simulink model "CoETS_TSEACo"  (R2016b)
settings: configuration reference "CodeGenConfigSet" (kept outside this file)
values from neighbouring files (symbols this model uses):
  CoETS_ctEngEmgcyRunCnt_C = Calibration.Parameter    [init_CoETS_TSEACo.m]
  CoETS_nTSCRmpSlopeNeg_C = Calibration.Parameter    [init_CoETS_TSEACo.m]
  CoETS_nTSCRmpSlopePos_C = Calibration.Parameter    [init_CoETS_TSEACo.m]
  CoETS_numTSEAPrioAE_C = Calibration.Parameter    [init_CoETS_TSEACo.m]
  CoETS_numTSEAPrioDE_C = Calibration.Parameter    [init_CoETS_TSEACo.m]
  CoETS_numTSEAPrioGpsLim_C = Calibration.Parameter    [init_CoETS_TSEACo.m]
  CoETS_numTSEAPrioPE_C = Calibration.Parameter    [init_CoETS_TSEACo.m]
  CoETS_numTSEAPrioTE_C = Calibration.Parameter    [init_CoETS_TSEACo.m]
  CoETS_numTSEAPrioVE_C = Calibration.Parameter    [init_CoETS_TSEACo.m]
  CoETS_stEngEmgcyRunEN_C = Calibration.Parameter    [init_CoETS_TSEACo.m]
  CoETS_stStartRelayCtrl_C = Calibration.Parameter    [init_CoETS_TSEACo.m]
  CoETS_stTboxUse_C = Calibration.Parameter    [init_CoETS_TSEACo.m]
  CoETS_stTSEATrqSpd_C = Calibration.Parameter    [init_CoETS_TSEACo.m]
  CoETS_swtTempSel_C = Calibration.Parameter    [init_CoETS_TSEACo.m]
  CoETS_tEngEmgcyRunTemp_C = Calibration.Parameter    [init_CoETS_TSEACo.m]
  CoETS_tiEngEmgcyRunTime_C = Calibration.Parameter    [init_CoETS_TSEACo.m]
  CoETS_tiEngEmgcyStartTime_C = Calibration.Parameter    [init_CoETS_TSEACo.m]
  CoETS_tiEngLockTime_C = Calibration.Parameter    [init_CoETS_TSEACo.m]
  CoETS_tiSetTimeTSEReq_CUR = Calibration.Parameter    [init_CoETS_TSEACo.m]
  CoETS_tiSetTimeTSEReq_CURX = Calibration.Parameter    [init_CoETS_TSEACo.m]
  CoETS_TrqTSCRmpSlopeNeg_C = Calibration.Parameter    [init_CoETS_TSEACo.m]
  CoETS_TrqTSCRmpSlopePos_C = Calibration.Parameter    [init_CoETS_TSEACo.m]
  Ecu_stGps_Status_C = Calibration.Parameter    [init_CoETS_TSEACo.m]
  EngPrt_nRateSp_C = Calibration.Parameter    [init_CoETS_TSEACo.m]
  Gps_nSpdLmt_C = Calibration.Parameter    [init_CoETS_TSEACo.m]
  TSC_nAEDes_C = Calibration.Parameter    [init_CoETS_TSEACo.m]
  TSC_nDEDes_C = Calibration.Parameter    [init_CoETS_TSEACo.m]
  TSC_nPEDes_C = Calibration.Parameter    [init_CoETS_TSEACo.m]
  TSC_nTEDes_C = Calibration.Parameter    [init_CoETS_TSEACo.m]
  TSC_nVEDes_C = Calibration.Parameter    [init_CoETS_TSEACo.m]
  TSC_rTrqAEDes_C = Calibration.Parameter    [init_CoETS_TSEACo.m]
  TSC_rTrqDEDes_C = Calibration.Parameter    [init_CoETS_TSEACo.m]
  TSC_rTrqPEDes_C = Calibration.Parameter    [init_CoETS_TSEACo.m]
  TSC_rTrqTEDes_C = Calibration.Parameter    [init_CoETS_TSEACo.m]
  TSC_rTrqVEDes_C = Calibration.Parameter    [init_CoETS_TSEACo.m]
  TSC_stAEErr_C = Calibration.Parameter    [init_CoETS_TSEACo.m]
  TSC_stAEMode_C = Calibration.Parameter    [init_CoETS_TSEACo.m]
  TSC_stDEErr_C = Calibration.Parameter    [init_CoETS_TSEACo.m]
  TSC_stDEMode_C = Calibration.Parameter    [init_CoETS_TSEACo.m]
  TSC_stModeBypassEN_C = Calibration.Parameter    [init_CoETS_TSEACo.m]
  TSC_stPEErr_C = Calibration.Parameter    [init_CoETS_TSEACo.m]
  TSC_stPEMode_C = Calibration.Parameter    [init_CoETS_TSEACo.m]
  TSC_stTEErr_C = Calibration.Parameter    [init_CoETS_TSEACo.m]
  TSC_stTEMode_C = Calibration.Parameter    [init_CoETS_TSEACo.m]
  TSC_stVEErr_C = Calibration.Parameter    [init_CoETS_TSEACo.m]
  TSC_stVEMode_C = Calibration.Parameter    [init_CoETS_TSEACo.m]
undefined symbols (not defined in the file or in its folder): CoETS_TSEACo_DT, EngState_conv, HLSDem_KpCorFac_MAPX, Switch_conv, TSC1_stSource_conv
libraries: simulink x82, CXLib x8
(part 1 of 2)
settings Model: Creator=Wollf  LastModifiedBy=xuxingpei
settings ConfigSetRef: SourceLocation=Base Workspace

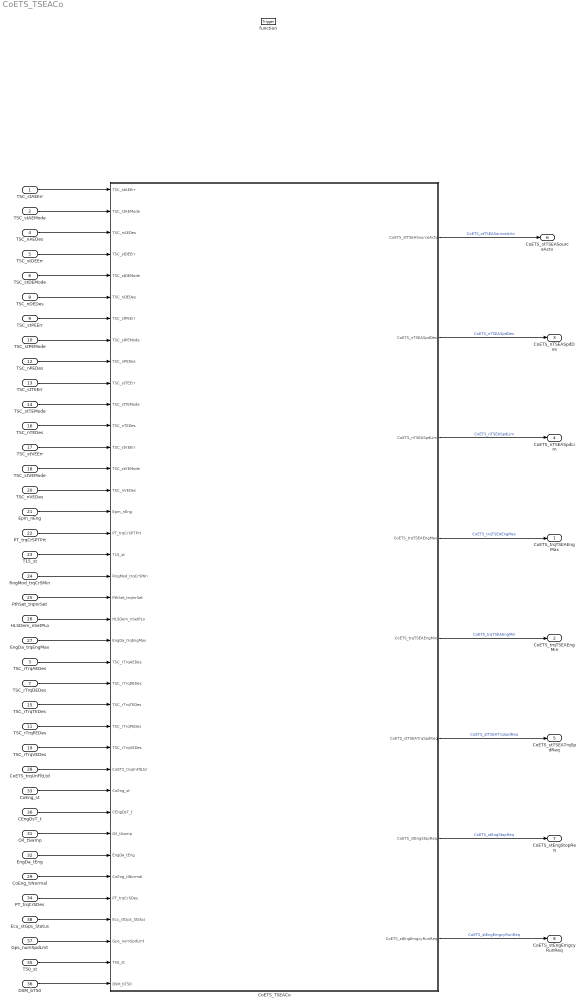
== system CoETS_TSEACo ==
  TSC_stAEErr : Inport  Description=Error status of receiving the TSC1-AE CAN message  OutMin=0  OutMax=1  OutDataTypeStr=State_uint8
  TSC_stAEMode : Inport  Description=Override control mode of TSC1-AE CAN message  Port=2  OutMin=0  OutMax=3  OutDataTypeStr=State_uint8
  TSC_rTrqAEDes : Inport  Description=|  Port=3  OutMin=0  OutMax=125  OutDataTypeStr=State_uint8
      | Requested torque percent / torque limit by TSC1-AE CAN
      | message Nm
  TSC_nAEDes : Inport  Tag=rpm  Description=Requested speed / speed limit by TSC1-AE message  Port=4  OutMin=0  OutMax=6000  OutDataTypeStr=EngSpeed_rpm
  TSC_stDEErr : Inport  Description=Error status of receiving the TSC1-DE CAN message  Port=5  OutMin=0  OutMax=1  OutDataTypeStr=State_uint8
  TSC_stDEMode : Inport  Description=Override control mode of TSC1-DE CAN message  Port=6  OutMin=0  OutMax=3  OutDataTypeStr=State_uint8
  TSC_rTrqDEDes : Inport  Description=|  Port=7  OutMin=0  OutMax=125  OutDataTypeStr=State_uint8
      | Requested torque percent/ torque limit by TSC1-DE CAN
      | message Nm
  TSC_nDEDes : Inport  Tag=rpm  Description=|  Port=8  OutMin=0  OutMax=8000  OutDataTypeStr=EngSpeed_rpm
      | Requested speed / speed limit by TSC1-DE CAN
      | message rpm
  TSC_stPEErr : Inport  Description=Error status of receiving the TSC1-PE CAN message  Port=9  OutMin=0  OutMax=1  OutDataTypeStr=State_uint8
  TSC_stPEMode : Inport  Description=Override control mode of TSC1-PE CAN message  Port=10  OutMin=0  OutMax=3  OutDataTypeStr=State_uint8
  TSC_rTrqPEDes : Inport  Description=|  Port=11  OutMin=0  OutMax=125  OutDataTypeStr=State_uint8
      | Requested torque percent/ torque limit by TSC1-PE CAN
      | message Nm
  TSC_nPEDes : Inport  Tag=rpm  Description=|  Port=12  OutMin=0  OutMax=8000  OutDataTypeStr=EngSpeed_rpm
      | Requested speed / speed limit by TSC1-PE CAN
      | message rpm
  TSC_stTEErr : Inport  Description=Error status of receiving the TSC1-TE CAN message  Port=13  OutMin=0  OutMax=1  OutDataTypeStr=State_uint8
  TSC_stTEMode : Inport  Description=Override control mode of TSC1-TE CAN message  Port=14  OutMin=0  OutMax=3  OutDataTypeStr=State_uint8
  TSC_rTrqTEDes : Inport  Description=|  Port=15  OutMin=0  OutMax=125  OutDataTypeStr=State_uint8
      | Requested torque percent / torque limit by TSC1-TE CAN
      | message Nm
  TSC_nTEDes : Inport  Tag=rpm  Description=|  Port=16  OutMin=0  OutMax=8000  OutDataTypeStr=EngSpeed_rpm
      | Requested speed / speed limit by TSC1-TE CAN
      | message rpm
  TSC_stVEErr : Inport  Description=Error status of receiving the TSC1-VE CAN message  Port=17  OutMin=0  OutMax=1  OutDataTypeStr=State_uint8
  TSC_stVEMode : Inport  Description=Override control mode of TSC1-VE CAN message.  Port=18  OutMin=0  OutMax=3  OutDataTypeStr=State_uint8
  TSC_rTrqVEDes : Inport  Description=|  Port=19  OutMin=0  OutMax=125  OutDataTypeStr=State_uint8
      | Requested torque percent/ torque limit by TSC1-VE CAN
      | message Nm
  TSC_nVEDes : Inport  Tag=rpm  Description=|  Port=20  OutMin=0  OutMax=8000  OutDataTypeStr=EngSpeed_rpm
      | Requested speed / speed limit by TSC1-VE CAN
      | message rpm
  Epm_nEng : Inport  Tag=rpm  Description=Engine speed  Port=21  OutMin=0  OutMax=6000  OutDataTypeStr=EngSpeed_rpm
  PT_trqCrSPTPrt : Inport  Tag=Nm  Description=Application parameter for powertrain protection train protection torque(crankshaft torque)  Port=22  OutMin=-3000  OutMax=3000  OutDataTypeStr=Trq_Nm
  T15_st : Inport  Description=Terminal 15 status after debouncing  Port=23  OutDataTypeStr=Enum: Switch_conv
  RngMod_trqCrSMin : Inport  Tag=Nm  Description=minimal crankshaft torque  Port=24  OutMin=-3276.8  OutMax=3276.7  OutDataTypeStr=Trq_Nm
  PthSet_trqInrSet : Inport  Tag=Nm  Description=Inner torque set value after monitoring limitation  Port=25  OutMin=-3000  OutMax=3276.7  OutDataTypeStr=Trq_Nm
  HLSDem_nSetPLo : Inport  Tag=rpm  Description=Minimum engine speed of HLSDem  Port=26  OutMin=0  OutMax=6000  OutDataTypeStr=EngSpeed_rpm
  EngDa_trqEngMax : Inport  Tag=Nm  Description=Maximum engine output torque  Port=27  OutMin=-3276.8  OutMax=3276.7  OutDataTypeStr=Trq_Nm
  CoETS_trqUnFltLtd : Inport  Tag=Nm  Description=Limited idle speed governor torque  Port=28  OutMin=-3276  OutMax=3276  OutDataTypeStr=Trq_Nm
  CoEng_tiNormal : Inport  Tag=ms  Description="Time since state\"CONENG_RUNNING\"was reached"  Port=29  OutMin=0  OutMax=42949672950  OutDataTypeStr=EngTime_ms
  CEngDsT_t : Inport  Tag=deg  Description=engine coolant temperature after filter  Port=30  OutMin=-200  OutMax=200  OutDataTypeStr=Temp_deg
  Oil_tSwmp : Inport  Tag=deg  Description=Oil temperature in oil sump  Port=31  OutMin=-50  OutMax=200  OutDataTypeStr=Temp_deg
  EngDa_tEng : Inport  Tag=deg  Description=Engine temperature  Port=32  OutMin=-1000  OutMax=1000  OutDataTypeStr=Temp_deg
  CoEng_st : Inport  Description=Engine coordinator state  Port=33  OutDataTypeStr=Enum: EngState_conv
  PT_trqCrSDes : Inport  Tag=Nm  Description=Application parameter for requested propulsion torque to engine(crankshaft torque)  Port=34  OutMin=-3000  OutMax=3000  OutDataTypeStr=Trq_Nm
  T50_st : Inport  Description=Terminal 50 status after debouncing  Port=35  OutDataTypeStr=Enum: Switch_conv
  DSM_bT50 : Inport  Description=DSM status from T50 switch  Port=36  OutMin=0  OutMax=1  OutDataTypeStr=boolean
  Gps_numSpdLmt : Inport  Description=Tbox speed limit original value  Port=37  OutMin=0  OutMax=65535  OutDataTypeStr=State_uint16
  Ecu_stGps_Status : Inport  Description=Tbox control status  Port=38  OutMin=0  OutMax=255  OutDataTypeStr=State_uint8
  function : TriggerPort  TriggerType=function-call  VariantControl=Variant
  CoETS_TSEACo : Subsystem
  CoETS_trqTSEAEngMax : Outport  Tag=Nm  Description=torque request to engine intervention decrement(Max)  OutMin=-3276  OutMax=3276  OutDataTypeStr=Trq_Nm
  CoETS_trqTSEAEngMin : Outport  Tag=Nm  Description=torque request to engine intervention increment(Min)  Port=2  OutMin=-3276  OutMax=3276  OutDataTypeStr=Trq_Nm
  CoETS_nTSEASpdDes : Outport  Tag=rpm  Description=|  Port=3  OutMin=0  OutMax=6000  OutDataTypeStr=EngSpeed_rpm
      | The desired/control engine speed requested from
      | TSC1 CAN messages. This desired/control engine
      | speed is given to the speed governor.
  CoETS_nTSEASpdLim : Outport  Tag=rpm  Description=|  Port=4  OutMin=0  OutMax=6000  OutDataTypeStr=EngSpeed_rpm
      | The engine speed limitation requested from TSC1
      | CAN messages. This engine speed limit is given to
      | the speed governor
  CoETS_stTSEATrqSpdReq : Outport  Description=Status of information about torque and speed intervention  Port=5  OutMin=0  OutMax=65535  OutDataTypeStr=State_uint16
  CoETS_stTSEASourceActv : Outport  Description=Status of information about source active  Port=6  OutDataTypeStr=Enum: TSC1_stSource_conv
  CoETS_stEngStopReq : Outport  Description=Tbox Engine stop request  Port=7  OutMin=0  OutMax=1  OutDataTypeStr=boolean
  CoETS_stEngEmgcyRunReq : Outport  Description=Tbox Engine emergency start request  Port=8  OutMin=0  OutMax=1  OutDataTypeStr=boolean
  wires:
  CoETS_TSEACo/4(CoETS_trqTSEAEngMax) -> CoETS_trqTSEAEngMax/1  "CoETS_trqTSEAEngMax"
  CoETS_TSEACo/5(CoETS_trqTSEAEngMin) -> CoETS_trqTSEAEngMin/1  "CoETS_trqTSEAEngMin"
  CoETS_TSEACo/2(CoETS_nTSEASpdDes) -> CoETS_nTSEASpdDes/1  "CoETS_nTSEASpdDes"
  CoETS_TSEACo/3(CoETS_nTSEASpdLim) -> CoETS_nTSEASpdLim/1  "CoETS_nTSEASpdLim"
  TSC_stAEErr/1 -> CoETS_TSEACo/1(TSC_stAEErr)
  TSC_stAEMode/1 -> CoETS_TSEACo/2(TSC_stAEMode)
  TSC_rTrqAEDes/1 -> CoETS_TSEACo/23(TSC_rTrqAEDes)
  TSC_nAEDes/1 -> CoETS_TSEACo/3(TSC_nAEDes)
  TSC_stDEErr/1 -> CoETS_TSEACo/4(TSC_stDEErr)
  TSC_stDEMode/1 -> CoETS_TSEACo/5(TSC_stDEMode)
  TSC_rTrqDEDes/1 -> CoETS_TSEACo/24(TSC_rTrqDEDes)
  TSC_nDEDes/1 -> CoETS_TSEACo/6(TSC_nDEDes)
  TSC_stPEErr/1 -> CoETS_TSEACo/7(TSC_stPEErr)
  TSC_stPEMode/1 -> CoETS_TSEACo/8(TSC_stPEMode)
  TSC_rTrqPEDes/1 -> CoETS_TSEACo/26(TSC_rTrqPEDes)
  TSC_nPEDes/1 -> CoETS_TSEACo/9(TSC_nPEDes)
  TSC_stTEErr/1 -> CoETS_TSEACo/10(TSC_stTEErr)
  TSC_stTEMode/1 -> CoETS_TSEACo/11(TSC_stTEMode)
  TSC_rTrqTEDes/1 -> CoETS_TSEACo/25(TSC_rTrqTEDes)
  TSC_nTEDes/1 -> CoETS_TSEACo/12(TSC_nTEDes)
  TSC_stVEErr/1 -> CoETS_TSEACo/13(TSC_stVEErr)
  TSC_stVEMode/1 -> CoETS_TSEACo/14(TSC_stVEMode)
  TSC_rTrqVEDes/1 -> CoETS_TSEACo/27(TSC_rTrqVEDes)
  TSC_nVEDes/1 -> CoETS_TSEACo/15(TSC_nVEDes)
  Epm_nEng/1 -> CoETS_TSEACo/16(Epm_nEng)
  PT_trqCrSPTPrt/1 -> CoETS_TSEACo/17(PT_trqCrSPTPrt)
  CoETS_TSEACo/6(CoETS_stTSEATrqSpdReq) -> CoETS_stTSEATrqSpdReq/1  "CoETS_stTSEATrqSpdReq"
  CoETS_TSEACo/1(CoETS_stTSEASourceActv) -> CoETS_stTSEASourceActv/1  "CoETS_stTSEASourceActv"
  T15_st/1 -> CoETS_TSEACo/18(T15_st)
  RngMod_trqCrSMin/1 -> CoETS_TSEACo/19(RngMod_trqCrSMin)
  PthSet_trqInrSet/1 -> CoETS_TSEACo/20(PthSet_trqInrSet)
  HLSDem_nSetPLo/1 -> CoETS_TSEACo/21(HLSDem_nSetPLo)
  EngDa_trqEngMax/1 -> CoETS_TSEACo/22(EngDa_trqEngMax)
  CoETS_trqUnFltLtd/1 -> CoETS_TSEACo/28(CoETS_trqUnFltLtd)
  CoEng_tiNormal/1 -> CoETS_TSEACo/33(CoEng_tiNormal)
  CEngDsT_t/1 -> CoETS_TSEACo/30(CEngDsT_t)
  CoEng_st/1 -> CoETS_TSEACo/29(CoEng_st)
  EngDa_tEng/1 -> CoETS_TSEACo/32(EngDa_tEng)
  Oil_tSwmp/1 -> CoETS_TSEACo/31(Oil_tSwmp)
  PT_trqCrSDes/1 -> CoETS_TSEACo/34(PT_trqCrSDes)
  CoETS_TSEACo/7(CoETS_stEngStopReq) -> CoETS_stEngStopReq/1  "CoETS_stEngStopReq"
  CoETS_TSEACo/8(CoETS_stEngEmgcyRunReq) -> CoETS_stEngEmgcyRunReq/1  "CoETS_stEngEmgcyRunReq"
  T50_st/1 -> CoETS_TSEACo/37(T50_st)
  DSM_bT50/1 -> CoETS_TSEACo/38(DSM_bT50)
  Gps_numSpdLmt/1 -> CoETS_TSEACo/36(Gps_numSpdLmt)
  Ecu_stGps_Status/1 -> CoETS_TSEACo/35(Ecu_stGps_Status)

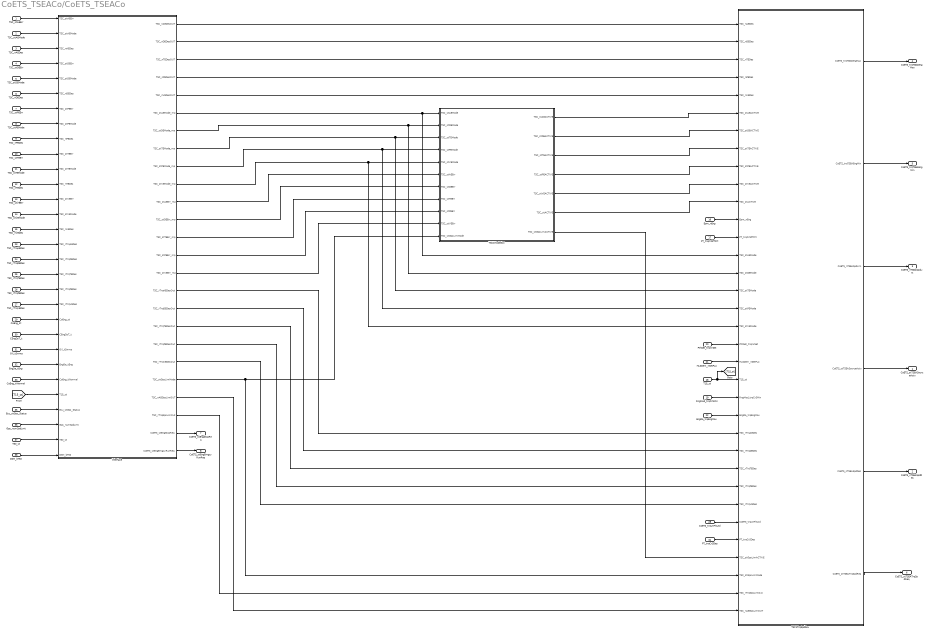
== system CoETS_TSEACo/CoETS_TSEACo ==
  TSC_stAEErr : Inport  Description=Error status of receiving the TSC1-AE CAN message  OutMin=0  OutMax=1  OutDataTypeStr=State_uint8
  TSC_stAEMode : Inport  Description=Override control mode of TSC1-AE CAN message  Port=2  OutMin=0  OutMax=3  OutDataTypeStr=State_uint8
  TSC_nAEDes : Inport  Tag=rpm  Description=Requested speed / speed limit by TSC1-AE message  Port=3  OutMin=0  OutMax=6000  OutDataTypeStr=EngSpeed_rpm
  TSC_stDEErr : Inport  Description=Error status of receiving the TSC1-DE CAN message  Port=4  OutMin=0  OutMax=1  OutDataTypeStr=State_uint8
  TSC_stDEMode : Inport  Description=Override control mode of TSC1-DE CAN message  Port=5  OutMin=0  OutMax=3  OutDataTypeStr=State_uint8
  TSC_nDEDes : Inport  Tag=rpm  Description=|  Port=6  OutMin=0  OutMax=8000  OutDataTypeStr=EngSpeed_rpm
      | Requested speed / speed limit by TSC1-DE CAN
      | message rpm
  TSC_stPEErr : Inport  Description=Error status of receiving the TSC1-PE CAN message  Port=7  OutMin=0  OutMax=1  OutDataTypeStr=State_uint8
  TSC_stPEMode : Inport  Description=Override control mode of TSC1-PE CAN message  Port=8  OutMin=0  OutMax=3  OutDataTypeStr=State_uint8
  TSC_nPEDes : Inport  Tag=rpm  Description=|  Port=9  OutMin=0  OutMax=8000  OutDataTypeStr=EngSpeed_rpm
      | Requested speed / speed limit by TSC1-PE CAN
      | message rpm
  TSC_stTEErr : Inport  Description=Error status of receiving the TSC1-TE CAN message  Port=10  OutMin=0  OutMax=1  OutDataTypeStr=State_uint8
  TSC_stTEMode : Inport  Description=Override control mode of TSC1-TE CAN message  Port=11  OutMin=0  OutMax=3  OutDataTypeStr=State_uint8
  TSC_nTEDes : Inport  Tag=rpm  Description=|  Port=12  OutMin=0  OutMax=8000  OutDataTypeStr=EngSpeed_rpm
      | Requested speed / speed limit by TSC1-TE CAN
      | message rpm
  TSC_stVEErr : Inport  Description=Error status of receiving the TSC1-VE CAN message  Port=13  OutMin=0  OutMax=1  OutDataTypeStr=State_uint8
  TSC_stVEMode : Inport  Description=Override control mode of TSC1-VE CAN message.  Port=14  OutMin=0  OutMax=3  OutDataTypeStr=State_uint8
  TSC_nVEDes : Inport  Tag=rpm  Description=|  Port=15  OutMin=0  OutMax=8000  OutDataTypeStr=EngSpeed_rpm
      | Requested speed / speed limit by TSC1-VE CAN
      | message rpm
  Epm_nEng : Inport  Tag=rpm  Description=Engine speed  Port=16  OutMin=0  OutMax=6000  OutDataTypeStr=EngSpeed_rpm
  PT_trqCrSPTPrt : Inport  Tag=Nm  Description=Application parameter for powertrain protection train protection torque(crankshaft torque)  Port=17  OutMin=-3000  OutMax=3000  OutDataTypeStr=Trq_Nm
  T15_st : Inport  Port=18
  RngMod_trqCrSMin : Inport  Port=19
  PthSet_trqInrSet : Inport  Port=20
  HLSDem_nSetPLo : Inport  Port=21
  EngDa_trqEngMax : Inport  Tag=Nm  Description=Maximum engine output torque  Port=22  OutMin=-3276.8  OutMax=3276.7  OutDataTypeStr=Trq_Nm
  TSC_rTrqAEDes : Inport  Description=|  Port=23  OutMin=0  OutMax=125  OutDataTypeStr=State_uint8
      | Requested torque percent / torque limit by TSC1-AE CAN
      | message Nm
  TSC_rTrqDEDes : Inport  Description=|  Port=24  OutMin=0  OutMax=125  OutDataTypeStr=State_uint8
      | Requested torque percent/ torque limit by TSC1-DE CAN
      | message Nm
  TSC_rTrqTEDes : Inport  Description=|  Port=25  OutMin=0  OutMax=125  OutDataTypeStr=State_uint8
      | Requested torque percent / torque limit by TSC1-TE CAN
      | message Nm
  TSC_rTrqPEDes : Inport  Description=|  Port=26  OutMin=0  OutMax=125  OutDataTypeStr=State_uint8
      | Requested torque percent/ torque limit by TSC1-PE CAN
      | message Nm
  TSC_rTrqVEDes : Inport  Description=|  Port=27  OutMin=0  OutMax=125  OutDataTypeStr=State_uint8
      | Requested torque percent/ torque limit by TSC1-VE CAN
      | message Nm
  CoETS_trqUnFltLtd : Inport  Port=28
  CoEng_st : Inport  Port=29
  CEngDsT_t : Inport  Tag=deg  Description=engine coolant temperature after filter  Port=30  OutMin=-200  OutMax=200  OutDataTypeStr=Temp_deg
  Oil_tSwmp : Inport  Tag=deg  Description=Oil temperature in oil sump  Port=31  OutMin=-50  OutMax=200  OutDataTypeStr=Temp_deg
  EngDa_tEng : Inport  Tag=deg  Description=Engine temperature  Port=32  OutMin=-1000  OutMax=1000  OutDataTypeStr=Temp_deg
  CoEng_tiNormal : Inport  Tag=ms  Description="Time since state\"CONENG_RUNNING\"was reached"  Port=33  OutMin=0  OutMax=42949672950  OutDataTypeStr=EngTime_ms
  PT_trqCrSDes : Inport  Tag=Nm  Description=Application parameter for requested propulsion torque to engine(crankshaft torque)  Port=34
  Ecu_stGps_Status : Inport  Port=35
  Gps_numSpdLmt : Inport  Port=36
  T50_st : Inport  Port=37
  DSM_bT50 : Inport  Port=38
  Interface : Subsystem
  TSC1ModeGov : Subsystem
  TSC1TrqSpdGov : Subsystem
  CoETS_stTSEASourceActv : Outport  Description=Identification name / number of the currently active EISGov client, which determines the current controller parameters
  CoETS_nTSEASpdDes : Outport  Tag=rpm  Description=|  Port=2  OutMin=0  OutMax=6000  OutDataTypeStr=EngSpeed_rpm
      | The desired/control engine speed requested from
      | TSC1 CAN messages. This desired/control engine
      | speed is given to the speed governor.
  CoETS_nTSEASpdLim : Outport  Tag=rpm  Description=|  Port=3  OutMin=0  OutMax=6000  OutDataTypeStr=EngSpeed_rpm
      | The engine speed limitation requested from TSC1
      | CAN messages. This engine speed limit is given to
      | the speed governor
  CoETS_trqTSEAEngMax : Outport  Tag=Nm  Description=torque request to engine intervention decrement(Max)  Port=4  OutMin=-3276  OutMax=3276  OutDataTypeStr=Trq_Nm
  CoETS_trqTSEAEngMin : Outport  Tag=Nm  Description=torque request to engine intervention increment(Min)  Port=5  OutMin=-3276  OutMax=3276  OutDataTypeStr=Trq_Nm
  CoETS_stTSEATrqSpdReq : Outport  Port=6
  CoETS_stEngStopReq : Outport  Port=7
  CoETS_stEngEmgcyRunReq : Outport  Port=8
  wires:
  PT_trqCrSPTPrt/1 -> TSC1TrqSpdGov/13(PT_trqCrSPTPrt)
  Epm_nEng/1 -> TSC1TrqSpdGov/12(Epm_nEng)
  TSC1TrqSpdGov/4(CoETS_stTSEASourceActv) -> CoETS_stTSEASourceActv/1
  TSC1TrqSpdGov/5(CoETS_nTSEASpdDes) -> CoETS_nTSEASpdDes/1
  TSC1TrqSpdGov/3(CoETS_nTSEASpdLim) -> CoETS_nTSEASpdLim/1
  TSC1TrqSpdGov/1(CoETS_trqTSEAEngMax) -> CoETS_trqTSEAEngMax/1
  TSC1TrqSpdGov/2(CoETS_trqTSEAEngMin) -> CoETS_trqTSEAEngMin/1
  T15_st/1 -> TSC1TrqSpdGov/21(T15_st), [T15_st]
  RngMod_trqCrSMin/1 -> TSC1TrqSpdGov/22(RngMod_trqCrSMin)
  PthSet_trqInrSet/1 -> TSC1TrqSpdGov/19(PthSet_trqInrSet)
  HLSDem_nSetPLo/1 -> TSC1TrqSpdGov/20(HLSDem_nSetPLo)
  EngDa_trqEngMax/1 -> TSC1TrqSpdGov/23(EngDa_trqEngMax)
  Interface/16(TSC_rTrqAEDesOut) -> TSC1TrqSpdGov/24(TSC_rTrqAEDes)
  Interface/17(TSC_rTrqDEDesOut) -> TSC1TrqSpdGov/25(TSC_rTrqDEDes)
  Interface/18(TSC_rTrqTEDesOut) -> TSC1TrqSpdGov/26(TSC_rTrqTEDes)
  Interface/19(TSC_rTrqPEDesOut) -> TSC1TrqSpdGov/27(TSC_rTrqPEDes)
  Interface/20(TSC_rTrqVEDesOut) -> TSC1TrqSpdGov/28(TSC_rTrqVEDes)
  Interface/1(TSC_nAEDesOUT) -> TSC1TrqSpdGov/1(TSC_nAEDes)
  Interface/2(TSC_nDEDesOUT) -> TSC1TrqSpdGov/2(TSC_nDEDes)
  Interface/3(TSC_nTEDesOUT) -> TSC1TrqSpdGov/3(TSC_nTEDes)
  Interface/4(TSC_nPEDesOUT) -> TSC1TrqSpdGov/4(TSC_nPEDes)
  Interface/5(TSC_nVEDesOUT) -> TSC1TrqSpdGov/5(TSC_nVEDes)
  CoETS_trqUnFltLtd/1 -> TSC1TrqSpdGov/29(CoETS_trqUnFltLtd)
  TSC1TrqSpdGov/6(CoETS_stTSEATrqSpdReq) -> CoETS_stTSEATrqSpdReq/1
  PT_trqCrSDes/1 -> TSC1TrqSpdGov/30(PT_trqCrSDes)
  TSC1ModeGov/1(TSC_stAEACTIVE) -> TSC1TrqSpdGov/6(TSC_stAEACTIVE)
  TSC1ModeGov/2(TSC_stDEACTIVE) -> TSC1TrqSpdGov/7(TSC_stDEACTIVE)
  TSC1ModeGov/3(TSC_stTEACTIVE) -> TSC1TrqSpdGov/8(TSC_stTEACTIVE)
  TSC1ModeGov/4(TSC_stPEACTIVE) -> TSC1TrqSpdGov/9(TSC_stPEACTIVE)
  TSC1ModeGov/5(TSC_stVEACTIVE) -> TSC1TrqSpdGov/10(TSC_stVEACTIVE)
  TSC1ModeGov/6(TSC_stACTIVE) -> TSC1TrqSpdGov/11(TSC_stACTIVE)
  Interface/11(TSC_stAEErr_mp) -> TSC1ModeGov/6(TSC_stAEErr)
  Interface/12(TSC_stDEErr_mp) -> TSC1ModeGov/7(TSC_stDEErr)
  Interface/13(TSC_stTEErr_mp) -> TSC1ModeGov/8(TSC_stTEErr)
  Interface/14(TSC_stPEErr_mp) -> TSC1ModeGov/9(TSC_stPEErr)
  Interface/15(TSC_stVEErr_mp) -> TSC1ModeGov/10(TSC_stVEErr)
  Interface/7(TSC_stDEMode_mp) -> TSC1TrqSpdGov/15(TSC_stDEMode), TSC1ModeGov/2(TSC_stDEMode)
  Interface/8(TSC_stTEMode_mp) -> TSC1TrqSpdGov/16(TSC_stTEMode), TSC1ModeGov/3(TSC_stTEMode)
  Interface/9(TSC_stPEMode_mp) -> TSC1TrqSpdGov/17(TSC_stPEMode), TSC1ModeGov/4(TSC_stPEMode)
  Interface/10(TSC_stVEMode_mp) -> TSC1TrqSpdGov/18(TSC_stVEMode), TSC1ModeGov/5(TSC_stVEMode)
  TSC_stAEErr/1 -> Interface/1(TSC_stAEErr)
  TSC_stAEMode/1 -> Interface/2(TSC_stAEMode)
  TSC_nAEDes/1 -> Interface/3(TSC_nAEDes)
  TSC_stDEErr/1 -> Interface/4(TSC_stDEErr)
  TSC_stDEMode/1 -> Interface/5(TSC_stDEMode)
  TSC_nDEDes/1 -> Interface/6(TSC_nDEDes)
  TSC_stPEErr/1 -> Interface/7(TSC_stPEErr)
  TSC_stPEMode/1 -> Interface/8(TSC_stPEMode)
  TSC_nPEDes/1 -> Interface/9(TSC_nPEDes)
  TSC_stTEErr/1 -> Interface/10(TSC_stTEErr)
  TSC_stTEMode/1 -> Interface/11(TSC_stTEMode)
  TSC_nTEDes/1 -> Interface/12(TSC_nTEDes)
  TSC_stVEErr/1 -> Interface/13(TSC_stVEErr)
  TSC_stVEMode/1 -> Interface/14(TSC_stVEMode)
  TSC_nVEDes/1 -> Interface/15(TSC_nVEDes)
  TSC_rTrqAEDes/1 -> Interface/16(TSC_rTrqAEDes)
  TSC_rTrqDEDes/1 -> Interface/17(TSC_rTrqDEDes)
  TSC_rTrqTEDes/1 -> Interface/18(TSC_rTrqTEDes)
  TSC_rTrqPEDes/1 -> Interface/19(TSC_rTrqPEDes)
  TSC_rTrqVEDes/1 -> Interface/20(TSC_rTrqVEDes)
  CoEng_st/1 -> Interface/21(CoEng_st)
  CEngDsT_t/1 -> Interface/22(CEngDsT_t)
  Oil_tSwmp/1 -> Interface/23(Oil_tSwmp)
  EngDa_tEng/1 -> Interface/24(EngDa_tEng)
  CoEng_tiNormal/1 -> Interface/25(CoEng_tiNormal)
  Interface/6(TSC_stAEMode_mp) -> TSC1TrqSpdGov/14(TSC_stAEMode), TSC1ModeGov/1(TSC_stAEMode)
  [T15_st] -> Interface/26(T15_st)
  TSC1ModeGov/7(TSC_stGpsLimACTIVE) -> TSC1TrqSpdGov/31(TSC_stGpsLimACTIVE)
  Interface/21(TSC_stGpsLimMode) -> TSC1TrqSpdGov/32(TSC_stGpsLimMode), TSC1ModeGov/11(TSC_stGpsLimMode)
  Interface/23(TSC_rTrqGpsLimOut) -> TSC1TrqSpdGov/33(TSC_rTrqGpsLimOut)
  Interface/22(TSC_nAEGpsLimOUT) -> TSC1TrqSpdGov/34(TSC_nAEGpsLimOUT)
  Interface/24(CoETS_stEngStopReq) -> CoETS_stEngStopReq/1
  Interface/25(CoETS_stEngEmgcyRunReq) -> CoETS_stEngEmgcyRunReq/1
  Gps_numSpdLmt/1 -> Interface/28(Gps_numSpdLmt)
  Ecu_stGps_Status/1 -> Interface/27(Ecu_stGps_Status)
  T50_st/1 -> Interface/29(T50_st)
  DSM_bT50/1 -> Interface/30(DSM_bT50)

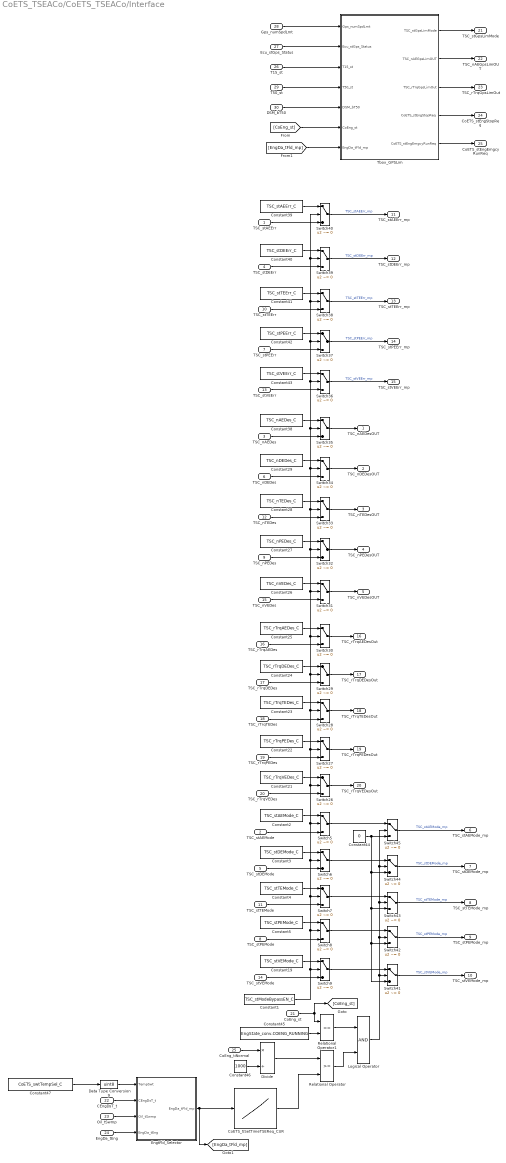
== system CoETS_TSEACo/CoETS_TSEACo/Interface ==
  TSC_stAEErr : Inport  Description=Error status of receiving the TSC1-AE CAN message  OutMin=0  OutMax=1  OutDataTypeStr=State_uint8
  TSC_stAEMode : Inport  Description=Override control mode of TSC1-AE CAN message  Port=2  OutMin=0  OutMax=3  OutDataTypeStr=State_uint8
  TSC_nAEDes : Inport  Tag=rpm  Description=Requested speed / speed limit by TSC1-AE message  Port=3  OutMin=0  OutMax=6000  OutDataTypeStr=EngSpeed_rpm
  TSC_stDEErr : Inport  Description=Error status of receiving the TSC1-DE CAN message  Port=4  OutMin=0  OutMax=1  OutDataTypeStr=State_uint8
  TSC_stDEMode : Inport  Description=Override control mode of TSC1-DE CAN message  Port=5  OutMin=0  OutMax=3  OutDataTypeStr=State_uint8
  TSC_nDEDes : Inport  Tag=rpm  Description=|  Port=6  OutMin=0  OutMax=8000  OutDataTypeStr=EngSpeed_rpm
      | Requested speed / speed limit by TSC1-DE CAN
      | message rpm
  TSC_stPEErr : Inport  Description=Error status of receiving the TSC1-PE CAN message  Port=7  OutMin=0  OutMax=1  OutDataTypeStr=State_uint8
  TSC_stPEMode : Inport  Description=Override control mode of TSC1-PE CAN message  Port=8  OutMin=0  OutMax=3  OutDataTypeStr=State_uint8
  TSC_nPEDes : Inport  Tag=rpm  Description=|  Port=9  OutMin=0  OutMax=8000  OutDataTypeStr=EngSpeed_rpm
      | Requested speed / speed limit by TSC1-PE CAN
      | message rpm
  TSC_stTEErr : Inport  Description=Error status of receiving the TSC1-TE CAN message  Port=10  OutMin=0  OutMax=1  OutDataTypeStr=State_uint8
  TSC_stTEMode : Inport  Description=Override control mode of TSC1-TE CAN message  Port=11  OutMin=0  OutMax=3  OutDataTypeStr=State_uint8
  TSC_nTEDes : Inport  Tag=rpm  Description=|  Port=12  OutMin=0  OutMax=8000  OutDataTypeStr=EngSpeed_rpm
      | Requested speed / speed limit by TSC1-TE CAN
      | message rpm
  TSC_stVEErr : Inport  Description=Error status of receiving the TSC1-VE CAN message  Port=13  OutMin=0  OutMax=1  OutDataTypeStr=State_uint8
  TSC_stVEMode : Inport  Description=Override control mode of TSC1-VE CAN message.  Port=14  OutMin=0  OutMax=3  OutDataTypeStr=State_uint8
  TSC_nVEDes : Inport  Tag=rpm  Description=|  Port=15  OutMin=0  OutMax=8000  OutDataTypeStr=EngSpeed_rpm
      | Requested speed / speed limit by TSC1-VE CAN
      | message rpm
  TSC_rTrqAEDes : Inport  Description=|  Port=16  OutMin=0  OutMax=125  OutDataTypeStr=State_uint8
      | Requested torque percent / torque limit by TSC1-AE CAN
      | message Nm
  TSC_rTrqDEDes : Inport  Description=|  Port=17  OutMin=0  OutMax=125  OutDataTypeStr=State_uint8
      | Requested torque percent/ torque limit by TSC1-DE CAN
      | message Nm
  TSC_rTrqTEDes : Inport  Description=|  Port=18  OutMin=0  OutMax=125  OutDataTypeStr=State_uint8
      | Requested torque percent / torque limit by TSC1-TE CAN
      | message Nm
  TSC_rTrqPEDes : Inport  Description=|  Port=19  OutMin=0  OutMax=125  OutDataTypeStr=State_uint8
      | Requested torque percent/ torque limit by TSC1-PE CAN
      | message Nm
  TSC_rTrqVEDes : Inport  Description=|  Port=20  OutMin=0  OutMax=125  OutDataTypeStr=State_uint8
      | Requested torque percent/ torque limit by TSC1-VE CAN
      | message Nm
  CoEng_st : Inport  Port=21
  CEngDsT_t : Inport  Tag=deg  Description=engine coolant temperature after filter  Port=22  OutMin=-200  OutMax=200  OutDataTypeStr=Temp_deg
  Oil_tSwmp : Inport  Tag=deg  Description=Oil temperature in oil sump  Port=23  OutMin=-50  OutMax=200  OutDataTypeStr=Temp_deg
  EngDa_tEng : Inport  Tag=deg  Description=Engine temperature  Port=24  OutMin=-1000  OutMax=1000  OutDataTypeStr=Temp_deg
  CoEng_tiNormal : Inport  Tag=ms  Description="Time since state\"CONENG_RUNNING\"was reached"  Port=25  OutMin=0  OutMax=42949672950  OutDataTypeStr=EngTime_ms
  T15_st : Inport  Port=26
  Ecu_stGps_Status : Inport  Port=27
  Gps_numSpdLmt : Inport  Port=28
  T50_st : Inport  Port=29
  DSM_bT50 : Inport  Port=30
  CoETS_tiSetTimeTSEReq_CUR : Lookup_n-D  NumberOfTableDimensions=1  BreakpointsForDimension1=CoETS_tiSetTimeTSEReq_CURX  BreakpointsForDimension2=HLSDem_KpCorFac_MAPX  Table=CoETS_tiSetTimeTSEReq_CUR  ExtrapMethod=Clip  InternalRulePriority=Speed  OutDataTypeStr=Inherit: Inherit via back propagation  RndMeth=Simplest  SaturateOnIntegerOverflow=on
  Constant1 : Constant  Value=TSC_stModeBypassEN_C
  Constant19 : Constant  Value=TSC_stVEMode_C
  Constant2 : Constant  Value=TSC_stAEMode_C
  Constant21 : Constant  Value=TSC_rTrqVEDes_C
  Constant22 : Constant  Value=TSC_rTrqPEDes_C
  Constant23 : Constant  Value=TSC_rTrqTEDes_C
  Constant24 : Constant  Value=TSC_rTrqDEDes_C
  Constant25 : Constant  Value=TSC_rTrqAEDes_C
  Constant26 : Constant  Value=TSC_nVEDes_C
  Constant27 : Constant  Value=TSC_nPEDes_C
  Constant28 : Constant  Value=TSC_nTEDes_C
  Constant29 : Constant  Value=TSC_nDEDes_C
  Constant3 : Constant  Value=TSC_stDEMode_C
  Constant38 : Constant  Value=TSC_nAEDes_C
  Constant39 : Constant  Value=TSC_stAEErr_C
  Constant4 : Constant  Value=TSC_stTEMode_C
  Constant40 : Constant  Value=TSC_stDEErr_C
  Constant41 : Constant  Value=TSC_stTEErr_C
  Constant42 : Constant  Value=TSC_stPEErr_C
  Constant43 : Constant  Value=TSC_stVEErr_C
  Constant44 : Constant  Value=0  OutDataTypeStr=Inherit: Inherit via back propagation
  Constant45 : Constant  Value=EngState_conv.COENG_RUNNING
  Constant46 : Constant  Value=1000  OutDataTypeStr=Inherit: Inherit via back propagation
  Constant47 : Constant  Value=CoETS_swtTempSel_C
  Constant5 : Constant  Value=TSC_stPEMode_C
  Data Type Conversion9 : DataTypeConversion  OutDataTypeStr=uint8
  Divide : Product  Inputs=*/  OutDataTypeStr=Inherit: Inherit via back propagation
  EngtFld_Selector : Subsystem
  Logical Operator : Logic  AllPortsSameDT=off  OutDataTypeStr=boolean
  Relational Operator : RelationalOperator  OutDataTypeStr=boolean  RndMeth=Simplest
  Relational Operator1 : RelationalOperator  Operator===  OutDataTypeStr=boolean  RndMeth=Nearest  InputSameDT=on
  Switch{5..9,26..45} (25 alike) : Switch  Criteria=u2 ~= 0
  Tbox_GPSLim : Subsystem
  TSC_nAEDesOUT : Outport
  TSC_nDEDesOUT : Outport  Port=2
  TSC_nTEDesOUT : Outport  Port=3
  TSC_nPEDesOUT : Outport  Port=4
  TSC_nVEDesOUT : Outport  Port=5
  TSC_stAEMode_mp : Outport  Port=6
  TSC_stDEMode_mp : Outport  Port=7
  TSC_stTEMode_mp : Outport  Port=8
  TSC_stPEMode_mp : Outport  Port=9
  TSC_stVEMode_mp : Outport  Port=10
  TSC_stAEErr_mp : Outport  Port=11
  TSC_stDEErr_mp : Outport  Port=12
  TSC_stTEErr_mp : Outport  Port=13
  TSC_stPEErr_mp : Outport  Port=14
  TSC_stVEErr_mp : Outport  Port=15
  TSC_rTrqAEDesOut : Outport  Port=16
  TSC_rTrqDEDesOut : Outport  Port=17
  TSC_rTrqTEDesOut : Outport  Port=18
  TSC_rTrqPEDesOut : Outport  Port=19
  TSC_rTrqVEDesOut : Outport  Port=20
  TSC_stGpsLimMode : Outport  Port=21
  TSC_nAEGpsLimOUT : Outport  Port=22
  TSC_rTrqGpsLimOut : Outport  Port=23
  CoETS_stEngStopReq : Outport  Port=24
  CoETS_stEngEmgcyRunReq : Outport  Port=25
  wires:
  TSC_stDEMode/1 -> Switch6/3
  Constant1/1 -> Switch27/2, Switch30/2, Switch40/2, Switch39/2, Switch38/2, Switch37/2, Switch36/2, Switch35/2, Switch34/2, Switch33/2, Switch32/2, Switch31/2, Switch29/2, Switch28/2, Switch26/2, Switch5/2, Switch6/2, Switch7/2, Switch8/2, Switch9/2
  Constant3/1 -> Switch6/1
  Constant4/1 -> Switch7/1
  TSC_stPEMode/1 -> Switch8/3
  Constant5/1 -> Switch8/1
  Constant19/1 -> Switch9/1
  TSC_stAEMode/1 -> Switch5/3
  TSC_stTEMode/1 -> Switch7/3
  TSC_stVEMode/1 -> Switch9/3
  TSC_rTrqVEDes/1 -> Switch26/3
  Constant2/1 -> Switch5/1
  Constant38/1 -> Switch35/1
  TSC_nVEDes/1 -> Switch31/3
  TSC_nTEDes/1 -> Switch33/3
  Constant26/1 -> Switch31/1
  TSC_nPEDes/1 -> Switch32/3
  TSC_rTrqAEDes/1 -> Switch30/3
  Constant22/1 -> Switch27/1
  Switch34/1 -> TSC_nDEDesOUT/1
  Switch33/1 -> TSC_nTEDesOUT/1
  Constant25/1 -> Switch30/1
  Switch29/1 -> TSC_rTrqDEDesOut/1
  Constant24/1 -> Switch29/1
  Constant29/1 -> Switch34/1
  Switch35/1 -> TSC_nAEDesOUT/1
  Switch30/1 -> TSC_rTrqAEDesOut/1
  TSC_rTrqPEDes/1 -> Switch27/3
  TSC_rTrqTEDes/1 -> Switch28/3
  TSC_rTrqDEDes/1 -> Switch29/3
  Constant23/1 -> Switch28/1
  Switch28/1 -> TSC_rTrqTEDesOut/1
  Constant21/1 -> Switch26/1
  Switch26/1 -> TSC_rTrqVEDesOut/1
  TSC_nDEDes/1 -> Switch34/3
  Switch27/1 -> TSC_rTrqPEDesOut/1
  TSC_nAEDes/1 -> Switch35/3
  Constant27/1 -> Switch32/1
  Constant28/1 -> Switch33/1
  Switch38/1 -> TSC_stTEErr_mp/1  "TSC_stTEErr_mp"
  TSC_stTEErr/1 -> Switch38/3
  Constant41/1 -> Switch38/1
  Switch8/1 -> Switch42/1
  TSC_stDEErr/1 -> Switch39/3
  Switch42/1 -> TSC_stPEMode_mp/1  "TSC_stPEMode_mp"
  Switch7/1 -> Switch43/1
  Switch37/1 -> TSC_stPEErr_mp/1  "TSC_stPEErr_mp"
  Switch43/1 -> TSC_stTEMode_mp/1  "TSC_stTEMode_mp"
  Switch6/1 -> Switch44/1
  Switch31/1 -> TSC_nVEDesOUT/1
  Switch40/1 -> TSC_stAEErr_mp/1  "TSC_stAEErr_mp"
  Switch44/1 -> TSC_stDEMode_mp/1  "TSC_stDEMode_mp"
  Constant40/1 -> Switch39/1
  Constant42/1 -> Switch37/1
  Constant43/1 -> Switch36/1
  Switch32/1 -> TSC_nPEDesOUT/1
  TSC_stVEErr/1 -> Switch36/3
  Switch39/1 -> TSC_stDEErr_mp/1  "TSC_stDEErr_mp"
  Switch36/1 -> TSC_stVEErr_mp/1  "TSC_stVEErr_mp"
  TSC_stAEErr/1 -> Switch40/3
  TSC_stPEErr/1 -> Switch37/3
  Switch9/1 -> Switch41/1
  Constant39/1 -> Switch40/1
  Switch41/1 -> TSC_stVEMode_mp/1  "TSC_stVEMode_mp"
  Switch5/1 -> Switch45/1
  Constant44/1 -> Switch45/3, Switch44/3, Switch43/3, Switch42/3, Switch41/3
  CoETS_tiSetTimeTSEReq_CUR/1 -> Relational Operator/2
  Relational Operator/1 -> Logical Operator/2
  Data Type Conversion9/1 -> EngtFld_Selector/1(TempSwt)
  Constant46/1 -> Divide/2
  Relational Operator1/1 -> Logical Operator/1
  CoEng_st/1 -> [CoEng_st], Relational Operator1/1
  Switch45/1 -> TSC_stAEMode_mp/1  "TSC_stAEMode_mp"
  CoEng_tiNormal/1 -> Divide/1
  EngDa_tEng/1 -> EngtFld_Selector/4(EngDa_tEng)
  Logical Operator/1 -> Switch42/2, Switch45/2, Switch44/2, Switch43/2, Switch41/2
  Constant45/1 -> Relational Operator1/2
  Constant47/1 -> Data Type Conversion9/1
  Oil_tSwmp/1 -> EngtFld_Selector/3(Oil_tSwmp)
  EngtFld_Selector/1(EngDa_tFld_mp) -> [EngDa_tFld_mp], CoETS_tiSetTimeTSEReq_CUR/1
  CEngDsT_t/1 -> EngtFld_Selector/2(CEngDsT_t)
  Divide/1 -> Relational Operator/1
  Gps_numSpdLmt/1 -> Tbox_GPSLim/1(Gps_numSpdLmt)
  Ecu_stGps_Status/1 -> Tbox_GPSLim/2(Ecu_stGps_Status)
  T15_st/1 -> Tbox_GPSLim/3(T15_st)
  T50_st/1 -> Tbox_GPSLim/4(T50_st)
  DSM_bT50/1 -> Tbox_GPSLim/5(DSM_bT50)
  Tbox_GPSLim/1(TSC_stGpsLimMode) -> TSC_stGpsLimMode/1
  Tbox_GPSLim/2(TSC_nAEGpsLimOUT) -> TSC_nAEGpsLimOUT/1
  Tbox_GPSLim/3(TSC_rTrqGpsLimOut) -> TSC_rTrqGpsLimOut/1
  Tbox_GPSLim/4(CoETS_stEngStopReq) -> CoETS_stEngStopReq/1
  Tbox_GPSLim/5(CoETS_stEngEmgcyRunReq) -> CoETS_stEngEmgcyRunReq/1
  [CoEng_st] -> Tbox_GPSLim/6(CoEng_st)
  [EngDa_tFld_mp] -> Tbox_GPSLim/7(EngDa_tFld_mp)

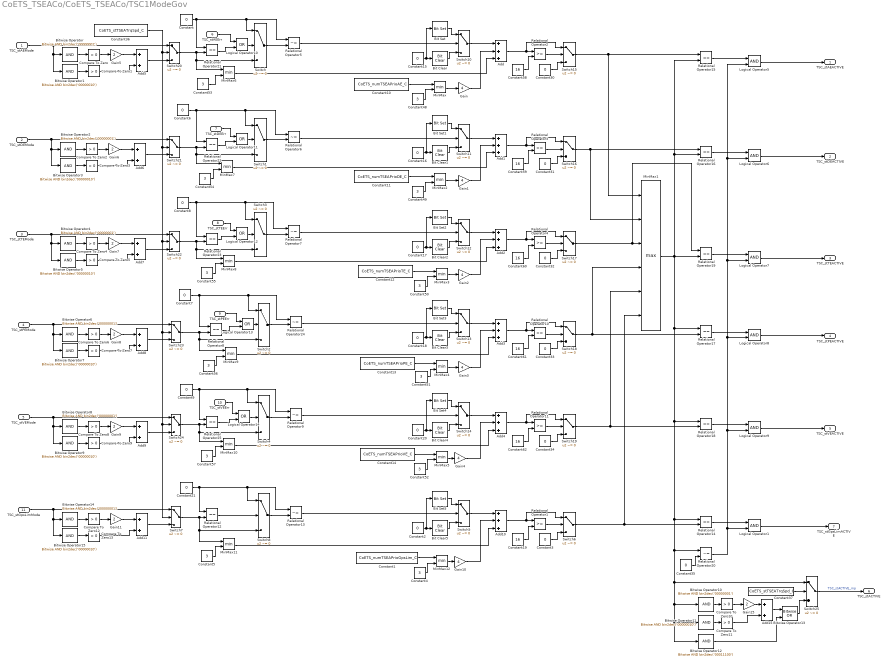
== system CoETS_TSEACo/CoETS_TSEACo/TSC1ModeGov ==
  TSC_stAEMode : Inport  Description=Override control mode of TSC1-AE CAN message  OutMin=0  OutMax=3  OutDataTypeStr=State_uint8
  TSC_stDEMode : Inport  Description=Override control mode of TSC1-DE CAN message  Port=2  OutMin=0  OutMax=3  OutDataTypeStr=State_uint8
  TSC_stTEMode : Inport  Description=Override control mode of TSC1-TE CAN message  Port=3  OutMin=0  OutMax=3  OutDataTypeStr=State_uint8
  TSC_stPEMode : Inport  Description=Override control mode of TSC1-PE CAN message  Port=4  OutMin=0  OutMax=3  OutDataTypeStr=State_uint8
  TSC_stVEMode : Inport  Description=Override control mode of TSC1-VE CAN message.  Port=5  OutMin=0  OutMax=3  OutDataTypeStr=State_uint8
  TSC_stAEErr : Inport  Description=Error status of receiving the TSC1-AE CAN message  Port=6  OutMin=0  OutMax=1  OutDataTypeStr=State_uint8
  TSC_stDEErr : Inport  Description=Error status of receiving the TSC1-DE CAN message  Port=7  OutMin=0  OutMax=1  OutDataTypeStr=State_uint8
  TSC_stTEErr : Inport  Description=Error status of receiving the TSC1-TE CAN message  Port=8  OutMin=0  OutMax=1  OutDataTypeStr=State_uint8
  TSC_stPEErr : Inport  Description=Error status of receiving the TSC1-PE CAN message  Port=9  OutMin=0  OutMax=1  OutDataTypeStr=State_uint8
  TSC_stVEErr : Inport  Description=Error status of receiving the TSC1-VE CAN message  Port=10  OutMin=0  OutMax=1  OutDataTypeStr=State_uint8
  TSC_stGpsLimMode : Inport  Description=Override control mode of TSC1-VE CAN message.  Port=11  OutMin=0  OutMax=3  OutDataTypeStr=State_uint8
  Add{,1..4,10} (6 alike) : Sum  Inputs=+++
  Add{5..9,11,15} (7 alike) : Sum
  Bit Clear{,1..5} (6 alike) : simulink/Logic and Bit Operations/Bit Clear  iBit=4
  Bit Set{,1..5} (6 alike) : simulink/Logic and Bit Operations/Bit Set  iBit=4
  Bitwise Operator{,2,4,6,8,10,14} (7 alike) : simulink/Logic and Bit Operations/Bitwise Operator  logicop=AND  UseBitMask=on  BitMask=bin2dec('00000001')  BitMaskRealWorld=Stored Integer
  Bitwise Operator{1,3,5,7,9,11,15} (7 alike) : simulink/Logic and Bit Operations/Bitwise Operator  logicop=AND  UseBitMask=on  BitMask=bin2dec('00000010')  BitMaskRealWorld=Stored Integer
  Bitwise Operator12 : simulink/Logic and Bit Operations/Bitwise Operator  logicop=AND  UseBitMask=on  BitMask=bin2dec('00011100')  BitMaskRealWorld=Stored Integer
  Bitwise Operator13 : simulink/Logic and Bit Operations/Bitwise Operator  logicop=OR  UseBitMask=off  NumInputPorts=2  BitMask=bin2dec('00011100')  BitMaskRealWorld=Stored Integer
  Compare To Zero{,1..13} (14 alike) : simulink/Logic and Bit Operations/Compare To Zero  relop=>  OutDataTypeStr=uint8
  Constant{,3,6..9,21,30..35} (13 alike) : Constant  Value=0  OutDataTypeStr=Inherit: Inherit via back propagation
  Constant1 : Constant  Value=CoETS_numTSEAPrioGpsLim_C
  Constant10 : Constant  Value=CoETS_numTSEAPrioAE_C
  Constant11 : Constant  Value=CoETS_numTSEAPrioDE_C
  Constant12 : Constant  Value=CoETS_numTSEAPrioTE_C
  Constant13 : Constant  Value=CoETS_numTSEAPrioPE_C
  Constant14 : Constant  Value=CoETS_numTSEAPrioVE_C
  Constant{2,15..18,20} (6 alike) : Constant  Value=0  OutDataTypeStr=uint8
  Constant{19,58..62} (6 alike) : Constant  Value=16  OutDataTypeStr=Inherit: Inherit via back propagation
  Constant36 : Constant  Value=CoETS_stTSEATrqSpd_C
  Constant37 : Constant  Value=CoETS_stTSEATrqSpd_C
  Constant{4..5,48..57} (12 alike) : Constant  Value=3  OutDataTypeStr=Inherit: Inherit via back propagation
  Gain{,1..4,10} (6 alike) : Gain  Gain=4  OutDataTypeStr=Inherit: Inherit via back propagation
  Gain{5..9,11,15} (7 alike) : Gain  Gain=2  OutDataTypeStr=Inherit: Inherit via back propagation
  Logical Operator{1,5..9} (6 alike) : Logic  AllPortsSameDT=off  OutDataTypeStr=boolean
  Logical Operator{10..14} (5 alike) : Logic  Operator=OR  AllPortsSameDT=off  OutDataTypeStr=boolean
  MinMax{,2..12} (12 alike) : MinMax  Inputs=2
  MinMax1 : MinMax  Function=max  Inputs=6
  Relational Operator{1..4,10..11} (6 alike) : RelationalOperator  OutDataTypeStr=boolean  RndMeth=Simplest
  Relational Operator{8,12,14..19,21..23,25} (12 alike) : RelationalOperator  Operator===  OutDataTypeStr=boolean  RndMeth=Simplest
  Relational Operator{5..7,9,13,20,24} (7 alike) : RelationalOperator  Operator=~=  OutDataTypeStr=boolean  RndMeth=Simplest
  Switch{,1..5,7..8,10..14,20..25} (19 alike) : Switch  Criteria=u2 ~= 0
  Switch{6,15..19} (6 alike) : Switch  Criteria=u2 ~= 0  Threshold=16
  TSC_stAEACTIVE : Outport
  TSC_stDEACTIVE : Outport  Port=2
  TSC_stTEACTIVE : Outport  Port=3
  TSC_stPEACTIVE : Outport  Port=4
  TSC_stVEACTIVE : Outport  Port=5
  TSC_stACTIVE : Outport  Port=6
  TSC_stGpsLimACTIVE : Outport  Port=7
  wires:
  Bit Set2/1 -> Switch12/1
  Constant9/1 -> Switch4/1, Relational Operator9/1, Relational Operator25/1
  Constant8/1 -> Relational Operator23/1, Switch3/1, Relational Operator7/1
  Bit Clear1/1 -> Switch11/3
  Relational Operator5/1 -> Switch10/2
  Bit Set4/1 -> Switch14/1
  Switch3/1 -> Relational Operator7/2
  Constant20/1 -> Bit Set4/1, Bit Clear4/1
  Relational Operator7/1 -> Switch12/2
  Bit Clear3/1 -> Switch13/3
  Bit Set1/1 -> Switch11/1
  Constant17/1 -> Bit Set2/1, Bit Clear2/1
  Bit Clear2/1 -> Switch12/3
  Constant18/1 -> Bit Set3/1, Bit Clear3/1
  Switch/1 -> Relational Operator5/2
  Constant/1 -> Relational Operator21/1, Switch/1, Relational Operator5/1
  Constant6/1 -> Relational Operator22/1, Switch1/1, Relational Operator6/1
  Bit Clear/1 -> Switch10/3
  Constant16/1 -> Bit Set1/1, Bit Clear1/1
  Bit Set3/1 -> Switch13/1
  Constant7/1 -> Switch2/1, Relational Operator24/1, Relational Operator8/1
  Bit Set/1 -> Switch10/1
  Constant15/1 -> Bit Set/1, Bit Clear/1
  Relational Operator6/1 -> Switch11/2
  Bit Clear4/1 -> Switch14/3
  Switch12/1 -> Add2/1
  Gain1/1 -> Add1/2
  Switch19/1 -> Relational Operator18/2, MinMax1/5
  Relational Operator20/1 -> Logical Operator1/2, Logical Operator9/2, Logical Operator8/2, Logical Operator6/2, Logical Operator5/2, Logical Operator7/2
  Switch15/1 -> Relational Operator15/1, MinMax1/1
  Relational Operator24/1 -> Switch13/2
  Relational Operator15/1 -> Logical Operator5/1
  Relational Operator9/1 -> Switch14/2
  Logical Operator7/1 -> TSC_stTEACTIVE/1
  Logical Operator5/1 -> TSC_stAEACTIVE/1
  Constant30/1 -> Switch15/3
  Logical Operator8/1 -> TSC_stPEACTIVE/1
  Logical Operator9/1 -> TSC_stVEACTIVE/1
  Gain4/1 -> Add4/2
  Switch13/1 -> Add3/1
  Switch16/1 -> Relational Operator16/1, MinMax1/2
  Relational Operator18/1 -> Logical Operator9/1
  Relational Operator16/1 -> Logical Operator6/1
  Logical Operator6/1 -> TSC_stDEACTIVE/1
  Switch18/1 -> Relational Operator17/2, MinMax1/4
  Constant35/1 -> Relational Operator20/2
  Gain/1 -> Add/2
  Relational Operator17/1 -> Logical Operator8/1
  Relational Operator19/1 -> Logical Operator7/1
  Constant10/1 -> MinMax/1
  Switch10/1 -> Add/1
  Gain3/1 -> Add3/2
  Gain2/1 -> Add2/2
  Switch17/1 -> MinMax1/3, Relational Operator19/1
  Switch11/1 -> Add1/1
  Switch14/1 -> Add4/1
  Bitwise Operator/1 -> Compare To Zero/1
  Relational Operator8/1 -> Logical Operator13/2
  Relational Operator25/1 -> Logical Operator14/2
  Logical Operator13/1 -> Switch2/2
  Logical Operator14/1 -> Switch4/2
  Switch2/1 -> Relational Operator24/2
  Logical Operator10/1 -> Switch/2
  Logical Operator12/1 -> Switch3/2
  Relational Operator21/1 -> Logical Operator10/2
  Switch4/1 -> Relational Operator9/2
  Relational Operator22/1 -> Logical Operator11/2
  Switch1/1 -> Relational Operator6/2
  Logical Operator11/1 -> Switch1/2
  Relational Operator23/1 -> Logical Operator12/2
  Switch25/1 -> TSC_stACTIVE/1  "TSC_stACTIVE_mp"
  Gain5/1 -> Add5/1
  Bitwise Operator13/1 -> Switch25/3
  Bitwise Operator1/1 -> Compare To Zero1/1
  Bitwise Operator11/1 -> Compare To Zero11/1
  MinMax1/1 -> Relational Operator15/2, Relational Operator16/2, Relational Operator14/1, Bitwise Operator10/1, Bitwise Operator11/1, Bitwise Operator12/1, Switch25/1, Relational Operator20/1, Relational Operator18/1, Relational Operator17/1, Relational Operator19/2
  Add5/1 -> Switch20/3
  Bitwise Operator10/1 -> Compare To Zero10/1
  Add6/1 -> Switch21/3
  Constant37/1 -> Switch25/2
  Bitwise Operator12/1 -> Bitwise Operator13/2
  TSC_stDEMode/1 -> Switch21/1, Bitwise Operator2/1, Bitwise Operator3/1
  Gain15/1 -> Add15/1
  Add15/1 -> Bitwise Operator13/1
  TSC_stAEErr/1 -> Logical Operator10/1
  TSC_stDEErr/1 -> Logical Operator11/1
  TSC_stTEErr/1 -> Logical Operator12/1
  TSC_stPEErr/1 -> Logical Operator13/1
  Bitwise Operator6/1 -> Compare To Zero6/1
  Add9/1 -> Switch24/3
  Bitwise Operator8/1 -> Compare To Zero8/1
  Bitwise Operator4/1 -> Compare To Zero4/1
  Gain9/1 -> Add9/1
  Bitwise Operator9/1 -> Compare To Zero9/1
  TSC_stTEMode/1 -> Switch22/1, Bitwise Operator4/1, Bitwise Operator5/1
  Compare To Zero8/1 -> Gain9/1
  Bitwise Operator3/1 -> Compare To Zero3/1
  Add7/1 -> Switch22/3
  Bitwise Operator7/1 -> Compare To Zero7/1
  Compare To Zero1/1 -> Add5/2
  Compare To Zero2/1 -> Gain6/1
  Gain8/1 -> Add8/1
  Compare To Zero9/1 -> Add9/2
  Bitwise Operator5/1 -> Compare To Zero5/1
  Compare To Zero4/1 -> Gain7/1
  Compare To Zero/1 -> Gain5/1
  TSC_stVEErr/1 -> Logical Operator14/1
  Bitwise Operator2/1 -> Compare To Zero2/1
  Compare To Zero5/1 -> Add7/2
  TSC_stAEMode/1 -> Bitwise Operator/1, Bitwise Operator1/1, Switch20/1
  Gain7/1 -> Add7/1
  Gain6/1 -> Add6/1
  TSC_stPEMode/1 -> Switch23/1, Bitwise Operator6/1, Bitwise Operator7/1
  Compare To Zero6/1 -> Gain8/1
  Compare To Zero7/1 -> Add8/2
  TSC_stVEMode/1 -> Switch24/1, Bitwise Operator8/1, Bitwise Operator9/1
  Compare To Zero3/1 -> Add6/2
  Add8/1 -> Switch23/3
  Compare To Zero10/1 -> Gain15/1
  Compare To Zero11/1 -> Add15/2
  Constant48/1 -> MinMax/2
  Constant11/1 -> MinMax2/1
  MinMax4/1 -> Gain3/1
  Constant52/1 -> MinMax5/2
  Constant49/1 -> MinMax2/2
  MinMax2/1 -> Gain1/1
  MinMax3/1 -> Gain2/1
  Constant51/1 -> MinMax4/2
  MinMax5/1 -> Gain4/1
  Constant14/1 -> MinMax5/1
  Switch20/1 -> MinMax6/1, Switch/3, Relational Operator21/2
  Constant53/1 -> MinMax6/2
  Constant12/1 -> MinMax3/1
  Constant50/1 -> MinMax3/2
  MinMax/1 -> Gain/1
  Constant13/1 -> MinMax4/1
  MinMax6/1 -> Add/3
  MinMax7/1 -> Add1/3
  Constant54/1 -> MinMax7/2
  Constant55/1 -> MinMax8/2
  MinMax8/1 -> Add2/3
  Switch23/1 -> Relational Operator8/2, MinMax9/1, Switch2/3
  Constant56/1 -> MinMax9/2
  Switch21/1 -> MinMax7/1, Switch1/3, Relational Operator22/2
  Switch22/1 -> Relational Operator23/2, MinMax8/1, Switch3/3
  Add1/1 -> Switch16/1, Relational Operator3/1
  Relational Operator4/1 -> Switch17/2
  Add4/1 -> Switch19/1, Relational Operator11/1
  Add3/1 -> Switch18/1, Relational Operator10/1
  Constant60/1 -> Relational Operator4/2
  Add/1 -> Switch15/1, Relational Operator2/1
  MinMax9/1 -> Add3/3
  Relational Operator11/1 -> Switch19/2
  Constant33/1 -> Switch18/3
  Constant32/1 -> Switch17/3
  Switch24/1 -> Relational Operator25/2, Switch4/3, MinMax10/1
  Constant59/1 -> Relational Operator3/2
  Relational Operator10/1 -> Switch18/2
  Constant58/1 -> Relational Operator2/2
  Constant34/1 -> Switch19/3
  Relational Operator2/1 -> Switch15/2
  Constant61/1 -> Relational Operator10/2
  Constant62/1 -> Relational Operator11/2
  Constant57/1 -> MinMax10/2
  Constant31/1 -> Switch16/3
  Relational Operator3/1 -> Switch16/2
  Add2/1 -> Switch17/1, Relational Operator4/1
  MinMax10/1 -> Add4/3
  Constant21/1 -> Switch8/1, Relational Operator13/1, Relational Operator12/1
  Bit Set5/1 -> Switch5/1
  Constant2/1 -> Bit Set5/1, Bit Clear5/1
  Bit Clear5/1 -> Switch5/3
  Relational Operator13/1 -> Switch5/2
  Gain10/1 -> Add10/2
  Switch5/1 -> Add10/1
  Relational Operator12/1 -> Switch8/2
  Switch8/1 -> Relational Operator13/2
  Constant36/1 -> Switch7/2, Switch24/2, Switch23/2, Switch22/2, Switch21/2, Switch20/2
  Add11/1 -> Switch7/3
  Bitwise Operator14/1 -> Compare To Zero12/1
  Gain11/1 -> Add11/1
  Bitwise Operator15/1 -> Compare To Zero13/1
  Compare To Zero12/1 -> Gain11/1
  Compare To Zero13/1 -> Add11/2
  TSC_stGpsLimMode/1 -> Bitwise Operator14/1, Bitwise Operator15/1, Switch7/1
  Constant4/1 -> MinMax12/2
  MinMax12/1 -> Gain10/1
  Constant1/1 -> MinMax12/1
  Add10/1 -> Switch6/1, Relational Operator1/1
  Relational Operator1/1 -> Switch6/2
  Switch7/1 -> Relational Operator12/2, Switch8/3, MinMax11/1
  Constant3/1 -> Switch6/3
  Constant19/1 -> Relational Operator1/2
  Constant5/1 -> MinMax11/2
  MinMax11/1 -> Add10/3
  Switch6/1 -> Relational Operator14/2, MinMax1/6
  Relational Operator14/1 -> Logical Operator1/1
  Logical Operator1/1 -> TSC_stGpsLimACTIVE/1
